simulink model "MARS"  (R2022a)
settings: Solver=VariableStepAuto  StartTime=0.0  StopTime=inf  RelTol=1e-3
model workspace (MAT data in the model file):
  T0 = -23.4
  h_trop = 7
  ingenuityParams : object (value not decoded)
symbols that are objects in the model workspace (value not decoded): ingenuityParams
undefined symbols (not defined in the file): body, collective1, collective2, duration, ingenuity, leg1, leg2, leg3, leg4, link_name, model_name, rotor1, rotor2, solarPanel, world_pose
libraries: fl_lib x35, robotgazebolib x31, nesl_utility x12, ee_lib x11, slpidlib x3, sharedtransform x2, simulink x1, shared6dof x1, aerolibwind2 x1
(part 3 of 3)

== stateflow chart MARS/M.A.R.S./Engine & Battery/System-Level Controls ==
  state Heating
    entry:
    heater = 1;
    fly = 0;
  state StandBy
    entry:
    heater = 0;
    fly = 0;
  state Land
    entry:
    heater = 0;
    fly = 1;
    during:
    altitudeRef = 0;
  state PrepareFlight
    entry:
    heater = 1;
    fly = 0;
  state Fly
    entry:
    heater = 0;
    fly = 1;
    during:
    altitudeRef = altitudeCom;
  (default) -> StandBy
  StandBy -> Heating [order 1] : [T < -15]
  Land -> StandBy : [altitude < 0.1]
  Heating -> StandBy : [T > -10 || SOC < 0.2]
  PrepareFlight -> StandBy [order 1] : [prepFlight == 0 || SOC <0.3]
  StandBy -> PrepareFlight [order 2] : [ prepFlight == 1 && SOC > 0.4]
  Fly -> Land : [prepFlight == 0 || SOC <0.3]
  PrepareFlight -> Fly [order 2] : [T>10]
  data: altitudeCom input; T input; SOC input; prepFlight input; heater output double; fly output; altitudeRef output; altitude input
